simulink model "gm_HDLPayloadScrambler_vs"  (R2022b)
settings: Solver=FixedStepDiscrete  StartTime=0.0  StopTime=stopTime  RelTol=1e-3
values from neighbouring files (symbols this model uses):
  fs = 1    [testPayloadScrambler.m]
undefined symbols (not defined in the file or in its folder): clk, clk_enable, reset_x
libraries: hdlsllib x23, dspsrcs4 x3, simulink x2, vivadosimlib x1
settings Model: Creator=cotti  LastModifiedBy=cotti
settings OptimizationCC: BlockReduction=off  ConditionallyExecuteInputs=off  DefaultParameterBehavior=Inlined  InheritOutputTypeSmallerThanSingle=on
settings DebuggingCC: AlgebraicLoopMsg=error  InheritedTsInSrcMsg=none  SingleTaskRateTransMsg=error
settings HardwareCC: ProdBitPerPointer=32  ProdBitPerSizeT=32  ProdBitPerPtrDiffT=32  ProdLargestAtomicFloat=None  ProdIntDivRoundTo=Undefined  ProdEndianess=Unspecified  ProdWordSize=32  ProdHWDeviceType=ASIC/FPGA->ASIC/FPGA  TargetBitPerLong=64  TargetBitPerPointer=64  TargetBitPerSizeT=64  TargetBitPerPtrDiffT=64  TargetLongLongMode=on  TargetIntDivRoundTo=Zero  TargetEndianess=LittleEndian  TargetWordSize=64  TargetHWDeviceType=Custom Processor->MATLAB Host Computer  ProdEqTarget=off

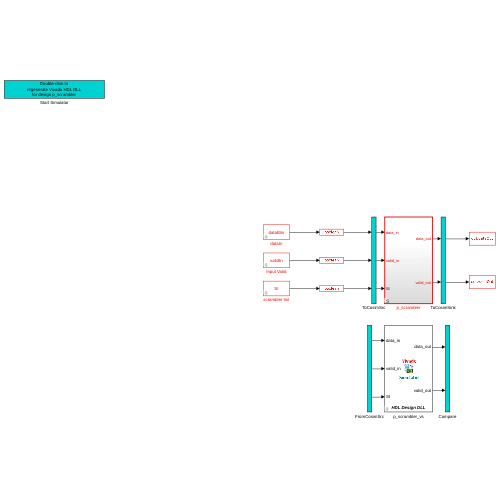
[thumbnail: Simulink's stored preview of the top-level diagram]
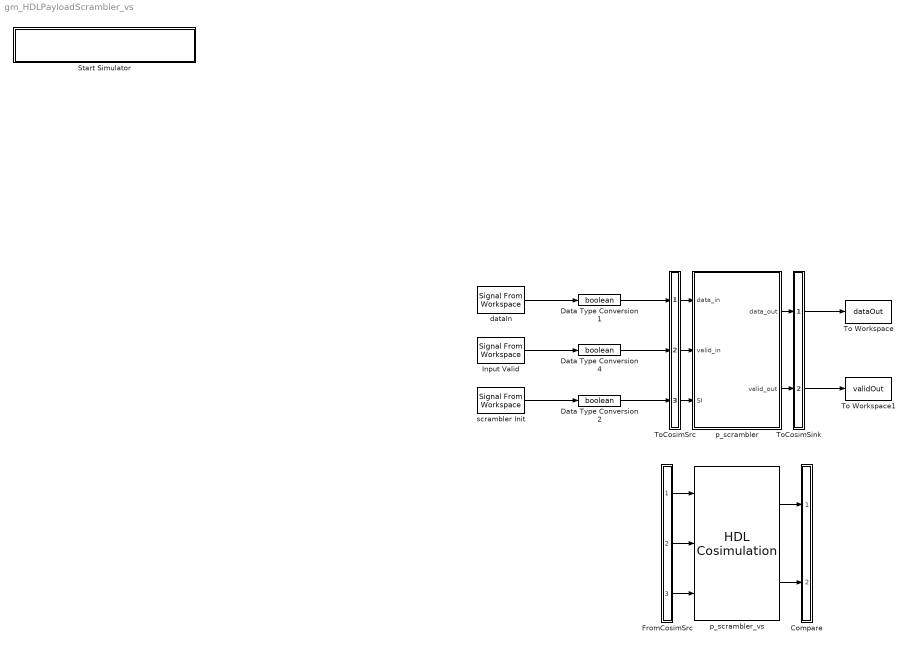
== system gm_HDLPayloadScrambler_vs ==
  Compare : Subsystem
      mask Display: disp('')
  Data Type Conversion1 : DataTypeConversion  OutDataTypeStr=boolean  SaturateOnIntegerOverflow=off  RndMeth=Floor
  Data Type Conversion2 : DataTypeConversion  OutDataTypeStr=boolean  SaturateOnIntegerOverflow=off  RndMeth=Floor
  Data Type Conversion4 : DataTypeConversion  OutDataTypeStr=boolean  SaturateOnIntegerOverflow=off  RndMeth=Floor
  FromCosimSrc : Subsystem
      mask Display: disp('')
  Input Valid : dspsrcs4/Signal From Workspace  X=validIn  Ts=1/fs  nsamps=1  OutputAfterFinalValue=Setting to zero  ignoreOrWarnInputAndFrameLengths=off  OutputFrames=off
  Start Simulator : Subsystem
      settings: OpenFcn=|
      | cosimDirName = pwd;
      | cd 'hdl_prj/hdlsrc/HDLPayloadScrambler';
      | [s,r] = system('vivado -mode batch -source gm_HDLPayloadScrambler_vs.tcl','-echo');
      | cd (cosimDirName);
      | clear cosimDirName;
      | if s
      |    error('Failed to create Vivado HDL design DLL using script gm_HDLPayloadScrambler_vs.tcl.');
      | end
      mask Display: disp('Double-click to\nregenerate Vivado HDL DLL\nfor design p_scrambler')
  To Workspace : ToWorkspace  VariableName=dataOut  SampleTime=1/fs
      settings: Save2DSignal=2-D array (concatenate along first dimension)
  To Workspace1 : ToWorkspace  VariableName=validOut  SampleTime=1/fs
      settings: Save2DSignal=2-D array (concatenate along first dimension)
  ToCosimSink : Subsystem
      mask Display: disp('')
  ToCosimSrc : Subsystem
      mask Display: disp('')
  dataIn : dspsrcs4/Signal From Workspace  X=dataBits  Ts=1/fs  nsamps=1  OutputAfterFinalValue=Setting to zero  ignoreOrWarnInputAndFrameLengths=off  OutputFrames=off
  p_scrambler : Subsystem
      settings: LibrarySourceBlock=|
      | hdlsllib/Ports &
      | Subsystems/Subsystem
  p_scrambler_vs : vivadosimlib/HDL Cosimulation  PortPaths=/p_scrambler/data_in;/p_scrambler/valid_in;/p_scrambler/SI;/p_scrambler/data_out;/p_scrambler/valid_out  PortModes=[1 1 1 2 2 ]  PortTimes=[-1 -1 -1 1 1 ]  PortSigns=[-1 -1 -1 0 0 ]  PortFracLengths=[0,0,0,0,0]  CommLocal=on  CommSharedMemory=on  CommPortNumber=4449  CommShowInfo=on  ClockPaths=clk;clk_enable;reset_x;  ClockModes=[2 4 3]  ClockTimes=[1e-08 3.7e-08 2.7e-08]  TclPostSimCommand="puts \"done\""  TimingMode=ns  TimingScaleFactor=10  idxCellArray={'UNUSED_VAR'}  CosimBypass=Full Simulation  AllowDirectFeedthrough=on  ProductName=EDA Simulator Link VS  RunAutoTimescale=off  HdlClocks=0  PreRunTime=40  PreRunTimeUnit=ns
  scrambler Init : dspsrcs4/Signal From Workspace  X=SI  Ts=1/fs  nsamps=1  OutputAfterFinalValue=Setting to zero  ignoreOrWarnInputAndFrameLengths=off  OutputFrames=off
  wires:
  dataIn/1 -> Data Type Conversion1/1
  Input Valid/1 -> Data Type Conversion4/1
  scrambler Init/1 -> Data Type Conversion2/1
  ToCosimSrc/1(out1) -> p_scrambler/1(data_in)
  ToCosimSrc/2(out2) -> p_scrambler/2(valid_in)
  ToCosimSrc/3(out3) -> p_scrambler/3(SI)
  p_scrambler/1(data_out) -> ToCosimSink/1(in1)
  p_scrambler/2(valid_out) -> ToCosimSink/2(in2)
  Data Type Conversion1/1 -> ToCosimSrc/1(in1)
  Data Type Conversion4/1 -> ToCosimSrc/2(in2)
  Data Type Conversion2/1 -> ToCosimSrc/3(in3)
  ToCosimSink/1(out1) -> To Workspace/1
  ToCosimSink/2(out2) -> To Workspace1/1
  FromCosimSrc/1(out1) -> p_scrambler_vs/1
  FromCosimSrc/2(out2) -> p_scrambler_vs/2
  FromCosimSrc/3(out3) -> p_scrambler_vs/3
  p_scrambler_vs/1 -> Compare/1(in1)
  p_scrambler_vs/2 -> Compare/2(in2)

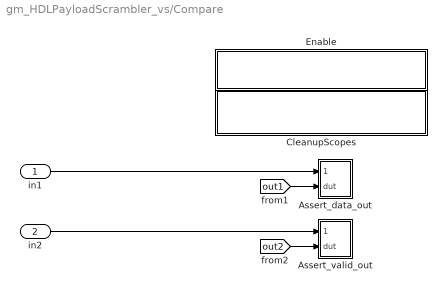
== system gm_HDLPayloadScrambler_vs/Compare ==
  in1 : Inport
  in2 : Inport  Port=2
  Assert_data_out : Subsystem
      settings: LibrarySourceBlock=hdlmdlgenlib/AssertEq
  Assert_valid_out : Subsystem
      settings: LibrarySourceBlock=hdlmdlgenlib/AssertEq
  CleanupScopes : Subsystem
      settings: OpenFcn=|
      | blkName = gcb; %self block
      | idx = regexp(blkName, '/CleanupScopes$', 'once');
      | blkParent = blkName(1:idx-1);
      | blks=find_system(blkParent, 'LookUnderMasks', 'all','blocktype', 'Scope');
      | for itr = 1:length(blks)
      | 	 hScopeCfg = get_param(blks{itr},'ScopeConfiguration');
      | 	 hScopeCfg.Visible = ~ hScopeCfg.Visible;
      | end
      | drawnow;
      mask Display: fprintf(message('hdlcoder:cosim:vnl_dblclick').getString());
  Enable : Subsystem
      settings: OpenFcn=|
      | blkName = gcb;
      | idx = regexp(blkName, '/Enable$', 'once');
      | blkParent = blkName(1:idx-1);
      | blks=find_system(blkParent, 'LookUnderMasks', 'all','blocktype', 'Assertion');
      | e = get_param(blks{1}, 'Enabled');
      | if strcmp(e, 'on'), f= 'off';, else, f = 'on';, end
      | for ii=1:length(blks), set_param(blks{ii}, 'Enabled', f);, end
      | set_param(gcb, 'MaskDisplay',['fprintf(message(''hdlcoder:cosim:vnl_dblclick_assertions'',','''',upper(e),'''',').getString())']);
      mask Display: fprintf(message('hdlcoder:cosim:vnl_dblclick_assertions','OFF').getString());
  wires:
  in1/1 -> Assert_data_out/1(cosim)
  [out1] -> Assert_data_out/2(dut)
  in2/1 -> Assert_valid_out/1(cosim)
  [out2] -> Assert_valid_out/2(dut)

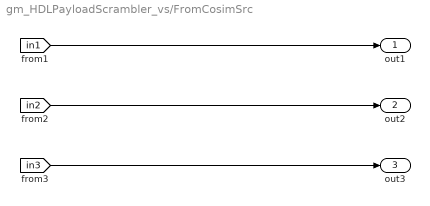
== system gm_HDLPayloadScrambler_vs/FromCosimSrc ==
  out1 : Outport
  out2 : Outport  Port=2
  out3 : Outport  Port=3
  wires:
  [in1] -> out1/1
  [in2] -> out2/1
  [in3] -> out3/1

== system gm_HDLPayloadScrambler_vs/Start Simulator ==

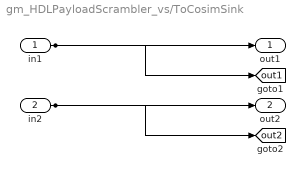
== system gm_HDLPayloadScrambler_vs/ToCosimSink ==
  in1 : Inport
  in2 : Inport  Port=2
  out1 : Outport
  out2 : Outport  Port=2
  tag scope: out1=global, out2=global
  wires:
  in1/1 -> out1/1, [out1]
  in2/1 -> out2/1, [out2]

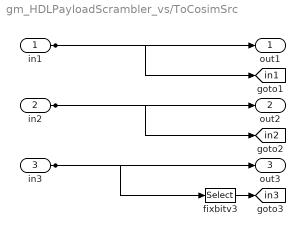
== system gm_HDLPayloadScrambler_vs/ToCosimSrc ==
  in1 : Inport
  in2 : Inport  Port=2
  in3 : Inport  Port=3
  fixbitv3 : Selector  IndexOptions=Index vector (dialog)  Indices=[4:-1:1]  OutputSizes=1
  out1 : Outport
  out2 : Outport  Port=2
  out3 : Outport  Port=3
  tag scope: in1=global, in2=global, in3=global
  wires:
  in1/1 -> out1/1, [in1]
  in2/1 -> out2/1, [in2]
  in3/1 -> out3/1, fixbitv3/1
  fixbitv3/1 -> [in3]

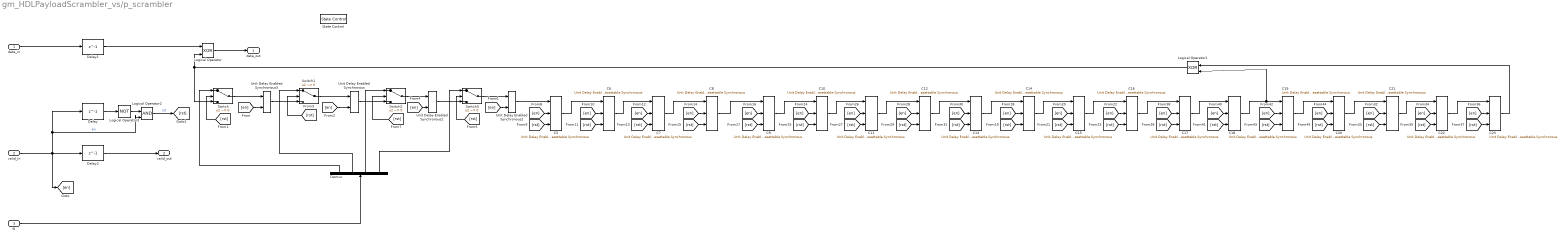
== system gm_HDLPayloadScrambler_vs/p_scrambler ==
  data_in : Inport
  valid_in : Inport  Port=2
  SI : Inport  Port=3
  C{5..23} (19 alike) : hdlsllib/Discrete/Unit Delay Enabled Resettable Synchronous  InitialCondition=1  SampleTime=-1
  Delay : Delay  DelayLength=1  InitialCondition=0  UseCircularBuffer=on
  Delay1 : Delay  DelayLength=1  InitialCondition=0  UseCircularBuffer=on
  Delay2 : Delay  DelayLength=1  InitialCondition=0  UseCircularBuffer=on
  Demux : Demux
  Logical Operator : Logic  Operator=XOR  IconShape=distinctive  AllPortsSameDT=off  OutDataTypeStr=boolean
  Logical Operator1 : Logic  Operator=XOR  IconShape=distinctive  AllPortsSameDT=off  OutDataTypeStr=boolean
  Logical Operator2 : Logic  IconShape=distinctive  AllPortsSameDT=off  OutDataTypeStr=boolean
  Logical Operator3 : Logic  Operator=NOT  IconShape=distinctive  AllPortsSameDT=off  OutDataTypeStr=boolean
  State Control : StateControl  StateControl=Synchronous
  Switch{,1..3} (4 alike) : Switch  Criteria=u2 ~= 0  OutDataTypeStr=boolean  SaturateOnIntegerOverflow=off  InputSameDT=off
  Unit Delay Enabled Synchronous{,1..3} (4 alike) : hdlsllib/Discrete/Unit Delay Enabled Synchronous  InitialCondition=1  SampleTime=-1
  data_out : Outport
  valid_out : Outport  Port=2  VectorParamsAs1DForOutWhenUnconnected=off
  wires:
  Logical Operator1/1 -> Switch/3, Logical Operator/2
  Logical Operator/1 -> data_out/1
  valid_in/1 -> Delay/1, Logical Operator2/2, Delay2/1, [en]  "en"
  data_in/1 -> Delay1/1
  Logical Operator2/1 -> [rst]  "rst"
  Logical Operator3/1 -> Logical Operator2/1
  Delay/1 -> Logical Operator3/1
  Delay1/1 -> Logical Operator/1
  Delay2/1 -> valid_out/1
  SI/1 -> Demux/1
  Demux/2 -> Switch1/1
  [en] -> Unit Delay Enabled Synchronous3/2
  [en] -> Unit Delay Enabled Synchronous/2
  [en] -> Unit Delay Enabled Synchronous1/2
  [en] -> Unit Delay Enabled Synchronous2/2
  [en] -> C5/2
  [en] -> C7/2
  [rst] -> C8/3
  C7/1 -> C8/1
  [rst] -> C7/3
  C5/1 -> C6/1
  [rst] -> C6/3
  [en] -> C8/2
  C6/1 -> C7/1
  [en] -> C6/2
  [rst] -> C5/3
  Unit Delay Enabled Synchronous2/1 -> C5/1
  C15/1 -> C16/1
  C9/1 -> C10/1
  [rst] -> C12/3
  [en] -> C16/2
  [rst] -> C11/3
  [en] -> C13/2
  C12/1 -> C13/1
  [rst] -> C10/3
  C10/1 -> C11/1
  [rst] -> C13/3
  [en] -> C11/2
  C14/1 -> C15/1
  [en] -> C9/2
  [en] -> C10/2
  [rst] -> C9/3
  C11/1 -> C12/1
  C13/1 -> C14/1
  [rst] -> C14/3
  [en] -> C12/2
  [rst] -> C16/3
  [en] -> C14/2
  [en] -> C15/2
  [rst] -> C15/3
  C8/1 -> C9/1
  [rst] -> C17/3
  [rst] -> C23/3
  C16/1 -> C17/1
  [en] -> C22/2
  C20/1 -> C21/1
  C18/1 -> Logical Operator1/2, C19/1
  [rst] -> C20/3
  [en] -> C23/2
  [en] -> C18/2
  [en] -> C19/2
  C22/1 -> C23/1
  C17/1 -> C18/1
  [rst] -> C21/3
  [rst] -> C19/3
  [en] -> C17/2
  [rst] -> C18/3
  C21/1 -> C22/1
  [en] -> C21/2
  [en] -> C20/2
  C19/1 -> C20/1
  [rst] -> C22/3
  C23/1 -> Logical Operator1/1
  [rst] -> Switch/2
  Demux/1 -> Switch/1
  Switch/1 -> Unit Delay Enabled Synchronous3/1
  Switch1/1 -> Unit Delay Enabled Synchronous/1
  [rst] -> Switch1/2
  Unit Delay Enabled Synchronous3/1 -> Switch1/3
  Switch2/1 -> Unit Delay Enabled Synchronous1/1
  Switch3/1 -> Unit Delay Enabled Synchronous2/1
  Unit Delay Enabled Synchronous1/1 -> Switch3/3
  [rst] -> Switch3/2
  Demux/4 -> Switch3/1
  Demux/3 -> Switch2/1
  Unit Delay Enabled Synchronous/1 -> Switch2/3
  [rst] -> Switch2/2

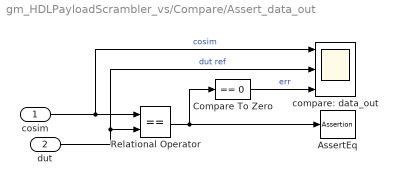
== system gm_HDLPayloadScrambler_vs/Compare/Assert_data_out ==
  cosim : Inport
  dut : Inport  Port=2
  AssertEq : Assertion  StopWhenAssertionFail=off
  Compare To Zero : simulink/Logic and Bit Operations/Compare To Zero  relop===  OutDataTypeStr=boolean
      settings: LibrarySourceBlock=|
      | hdlmdlgenlib/AssertEq/Compare
      | To Zero
  Relational Operator : RelationalOperator  Operator===  OutDataTypeStr=boolean  InputSameDT=off
  compare: data_out : Scope  NumInputPorts=3
  wires:
  Compare To Zero/1 -> compare: data_out/3  "err"
  Relational Operator/1 -> Compare To Zero/1, AssertEq/1
  cosim/1 -> compare: data_out/1, Relational Operator/1  "cosim"
  dut/1 -> compare: data_out/2, Relational Operator/2  "dut ref"

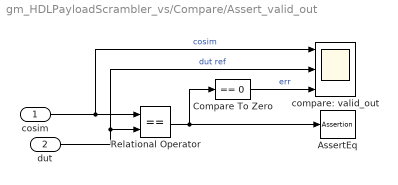
== system gm_HDLPayloadScrambler_vs/Compare/Assert_valid_out ==
  cosim : Inport
  dut : Inport  Port=2
  AssertEq : Assertion  StopWhenAssertionFail=off
  Compare To Zero : simulink/Logic and Bit Operations/Compare To Zero  relop===  OutDataTypeStr=boolean
      settings: LibrarySourceBlock=|
      | hdlmdlgenlib/AssertEq/Compare
      | To Zero
  Relational Operator : RelationalOperator  Operator===  OutDataTypeStr=boolean  InputSameDT=off
  compare: valid_out : Scope  NumInputPorts=3
  wires:
  Compare To Zero/1 -> compare: valid_out/3  "err"
  Relational Operator/1 -> Compare To Zero/1, AssertEq/1
  cosim/1 -> compare: valid_out/1, Relational Operator/1  "cosim"
  dut/1 -> compare: valid_out/2, Relational Operator/2  "dut ref"

== system gm_HDLPayloadScrambler_vs/Compare/CleanupScopes ==

== system gm_HDLPayloadScrambler_vs/Compare/Enable ==
